simulink model "Simple_L_battery_single"  (R2020a)
settings: Solver=VariableStepAuto  StartTime=0.0  StopTime=10.0  MaxStep=1e-2  RelTol=1e-3
undefined symbols (not defined in the file): CQ, I, Ke, Om, R, Ra, speedCmd, V0
libraries: simulink x1, fmu_me_lib x1
settings Model: Creator=Bob  LastModifiedBy=meagh
settings SFSimCC: CustomCodeUndefinedFunction=UseInterfaceOnly

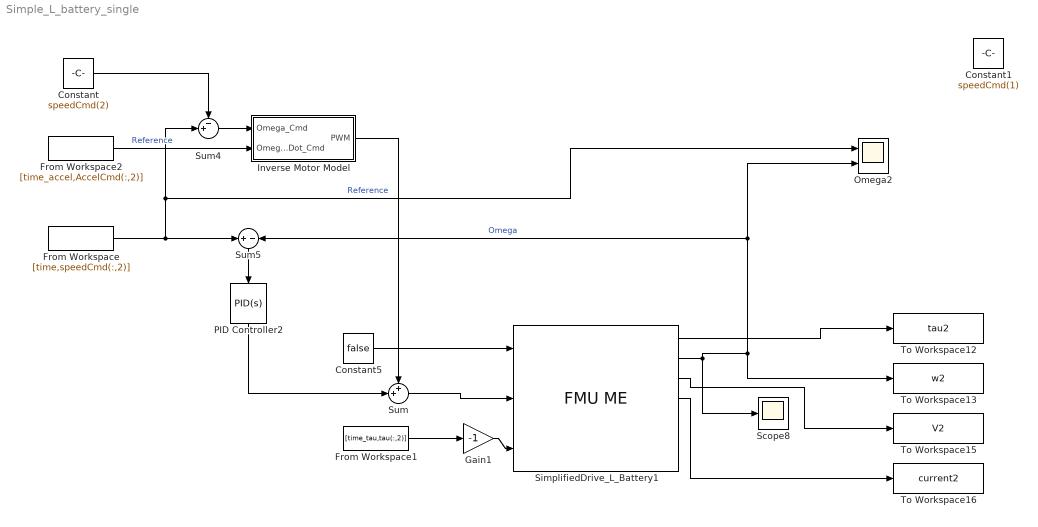
== system Simple_L_battery_single ==
  Constant : Constant  Value=speedCmd(2)
  Constant1 : Constant  Value=speedCmd(1)
  Constant5 : Constant  Value=false  OutDataTypeStr=boolean
  From Workspace : FromWorkspace  VariableName=[time,speedCmd(:,2)]
  From Workspace1 : FromWorkspace  VariableName=[time_tau,tau(:,2)]
  From Workspace2 : FromWorkspace  VariableName=[time_accel,AccelCmd(:,2)]
  Gain1 : Gain  Gain=-1
  Inverse Motor Model : Subsystem
  Omega2 : Scope  NumInputPorts=2
  PID Controller2 : simulink/Continuous/PID Controller  Controller=PID  Form=Parallel  TimeDomain=Continuous-time  UseExternalTs=off  SampleTime=-1  IntegratorMethod=Forward Euler  FilterMethod=Forward Euler  ControllerParametersSource=internal  P=0.0184*0.2  I=0.0184  D=0  UseFilter=on  N=100  TunerSelectOption=Transfer Function Based (PID Tuner App)  InitialConditionSource=internal  InitialConditionForIntegrator=0  InitialConditionForFilter=0  DifferentiatorICPrevScaledInput=0  ExternalReset=none  TrackingMode=off  Kt=1  LimitOutput=off  UpperSaturationLimit=inf  LowerSaturationLimit=-inf  LinearizeAsGain=on  AntiWindupMode=none  Kb=1  POutMin=[]  POutMax=[]  IOutMin=[]  IOutMax=[]  DOutMin=[]  DOutMax=[]  NOutMin=[]  NOutMax=[]  SumOutMin=[]  SumOutMax=[]  SaturationOutMin=[]  SaturationOutMax=[]  PParamMin=[]  PParamMax=[]  IParamMin=[]  IParamMax=[]  DParamMin=[]  DParamMax=[]  NParamMin=[]  NParamMax=[]  KbParamMin=[]  KbParamMax=[]  KtParamMin=[]  KtParamMax=[]  KbOutMin=[]  KbOutMax=[]  KtOutMin=[]  KtOutMax=[]  IntegratorOutMin=[]  IntegratorOutMax=[]  FilterOutMin=[]  FilterOutMax=[]  SumI1OutMin=[]  SumI1OutMax=[]  SumI2OutMin=[]  SumI2OutMax=[]  SumI3OutMin=[]  SumI3OutMax=[]  SumI4OutMin=[]  SumI4OutMax=[]  SumDOutMin=[]  SumDOutMax=[]  DifferentiatorOutMin=[]  DifferentiatorOutMax=[]  FilterDiffOutCoefMin=[]  FilterDiffOutCoefMax=[]  ReciprocalOutMin=[]  ReciprocalOutMax=[]  SumDenOutMin=[]  SumDenOutMax=[]  SumNumOutMin=[]  SumNumOutMax=[]  DivideOutMin=[]  DivideOutMax=[]  UdiffTsProdOutMin=[]  UdiffTsProdOutMax=[]  NTsProdOutMin=[]  NTsProdOutMax=[]  UintegralTsProdOutMin=[]  UintegralTsProdOutMax=[]  UngainTsProdOutMin=[]  UngainTsProdOutMax=[]  IntegratorContinuousStateAttributes=''  IntegratorStateMustResolveToSignalObject=off  IntegratorRTWStateStorageClass=Auto  FilterContinuousStateAttributes=''  FilterStateMustResolveToSignalObject=off  FilterRTWStateStorageClass=Auto  ParallelPVariant=InternalParameters  IdealPVariant=Disabled  IVariant=InternalParameters  DVariant=InternalParameters  IntegratorVariant=Continuous  SatVariant=Disabled  AWVariant=Passthrough  PCopyVariant=Disabled  TRVariant=Disabled  FdbkBlocksVariant=Forward  IdealPFdbkVariant=Disabled  SatFdbkVariant=Disabled  DerivativeFilterVariant=ContFilter  NVariant=InternalParameters  NCopyVariant=Disabled  FilterICVariant=InternalICsFilter  IntegratorICVariant=InternalICs  ExternalResetVariant=Disabled  TRSumVariant=Passthrough  SumFdbkVariant=Disabled  SumVariant=Sum_PID  TsampFilterVariant=InternalTs  TsampNgainVariant=Passthrough  TsampIntegralVariant=Passthrough
  Scope8 : Scope
  SimplifiedDrive_L_Battery1 : fmu_me_lib/FMU ME  Description=Simulates an FMU for Model Exchange 1.0 or Model Exchange 2.0.  dummy=0
  Sum : Sum  Inputs=++|
  Sum4 : Sum  Inputs=-+|
  Sum5 : Sum  Inputs=+|-
  To Workspace12 : ToWorkspace  VariableName=tau2  SaveFormat=Timeseries  SampleTime=-1
  To Workspace13 : ToWorkspace  VariableName=w2  SaveFormat=Timeseries  SampleTime=-1
  To Workspace15 : ToWorkspace  VariableName=V2  SaveFormat=Timeseries  SampleTime=-1
  To Workspace16 : ToWorkspace  VariableName=current2  SaveFormat=Timeseries  SampleTime=-1
  wires:
  Constant5/1 -> SimplifiedDrive_L_Battery1/1
  SimplifiedDrive_L_Battery1/1 -> To Workspace12/1
  SimplifiedDrive_L_Battery1/4 -> To Workspace16/1
  SimplifiedDrive_L_Battery1/3 -> To Workspace15/1
  SimplifiedDrive_L_Battery1/2 -> To Workspace13/1, Sum5/2, Omega2/2, Scope8/1  "Omega"
  Sum5/1 -> PID Controller2/1
  From Workspace1/1 -> Gain1/1
  Gain1/1 -> SimplifiedDrive_L_Battery1/3
  From Workspace/1 -> Omega2/1, Sum4/2, Sum5/1  "Reference"
  From Workspace2/1 -> Inverse Motor Model/2(OmegaDot_Cmd)  "Reference"
  PID Controller2/1 -> Sum/2
  Sum/1 -> SimplifiedDrive_L_Battery1/2
  Inverse Motor Model/1(PWM) -> Sum/1
  Sum4/1 -> Inverse Motor Model/1(Omega_Cmd)
  Constant/1 -> Sum4/1

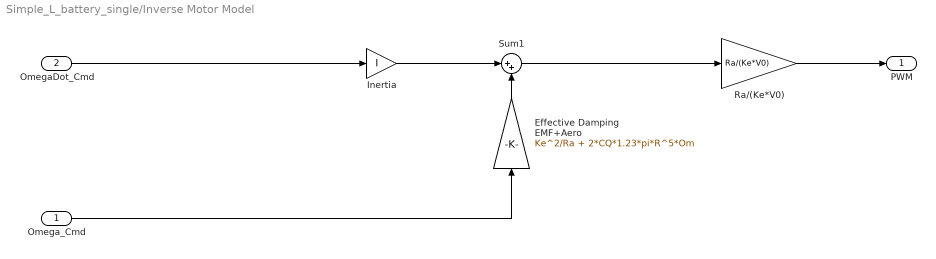
== system Simple_L_battery_single/Inverse Motor Model ==
  Omega_Cmd : Inport
  OmegaDot_Cmd : Inport  Port=2
  Effective Damping EMF+Aero : Gain  Gain=Ke^2/Ra + 2*CQ*1.23*pi*R^5*Om
  Inertia : Gain  Gain=I
  Ra/(Ke*V0) : Gain  Gain=Ra/(Ke*V0)
  Sum1 : Sum  Inputs=|++
  PWM : Outport  VectorParamsAs1DForOutWhenUnconnected=off
  wires:
  Ra/(Ke*V0)/1 -> PWM/1
  Sum1/1 -> Ra/(Ke*V0)/1
  Effective Damping EMF+Aero/1 -> Sum1/2
  Inertia/1 -> Sum1/1
  Omega_Cmd/1 -> Effective Damping EMF+Aero/1
  OmegaDot_Cmd/1 -> Inertia/1
